simulink model "A1_finalized"  (R2024a)
settings: Solver=FixedStepAuto  StartTime=0.0  StopTime=10.0  FixedStep=1e-3  RelTol=1e-3  EnableMultiTasking=on
undefined symbols (not defined in the file): D0, D1, D10, D11, D12, D13, D2, D3, D4, D5, D6, D7, D8, D9, PTA0, PTA1, PTA2, PTB23, PTB9, PTC16, PTC17, PTC2, PTC3, PTC4, PTD0, PTD1, PTD2, PTD3
libraries: frdmk64flib x17
settings Model: ExtModeTrigDuration=5  Creator=haani  LastModifiedBy=hmz04
settings OptimizationCC: EnhancedBackFolding=on  PassReuseOutputArgsAs=Individual arguments  ZeroExternalMemoryAtStartup=off  ZeroInternalMemoryAtStartup=off  MaxStackSize=64  OptimizeBlockOrder=speed  DifferentSizesBufferReuse=on  OptimizationCustomize=off  EfficientTunableParamExpr=on
settings DebuggingCC: ParameterTunabilityLossMsg=error
settings HardwareCC: ProdBitPerPointer=32  ProdBitPerSizeT=32  ProdBitPerPtrDiffT=32  ProdLargestAtomicInteger=Long  ProdLargestAtomicFloat=Double  ProdWordSize=32  ProdHWDeviceType=ARM Compatible->ARM Cortex
settings SFSimCC: MATLABDynamicMemAlloc=off
settings RTWCC: Description=Embedded Coder  SystemTargetFile=ert.tlc  HardwareBoard=NXP FRDM-K64F  TLCOptions="-aInlineSetEventsForThisBaseRateFcn=TLC_FALSE -aSuppressMultiTaskScheduler=TLC_FALSE  -aRateBasedStepFcn=0"  TemplateMakefile=ert_default_tmf  Toolchain=GNU Tools for ARM Embedded Processors
settings CodeAppCC: ForceParamTrailComments=on  IgnoreCustomStorageClasses=off  OperatorAnnotations=on  SimulinkDataObjDesc=on  SFDataObjDesc=on  InsertBlockDesc=on
settings ERTTargetCC: ExtModeTransport=4  ExtModeMexFile=sendToCommService

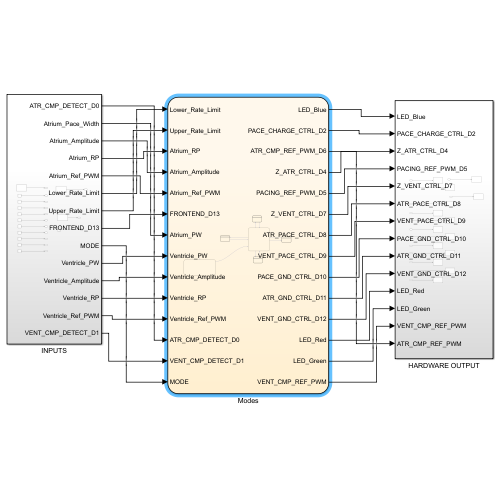
[thumbnail: Simulink's stored preview of the top-level diagram]
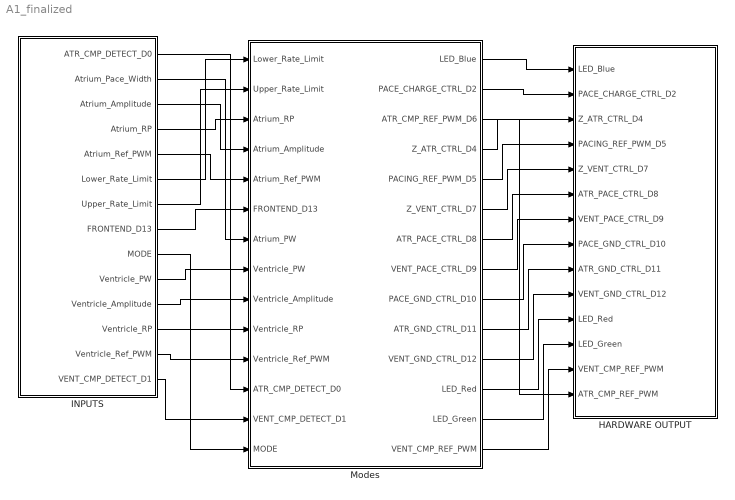
== system A1_finalized ==
  HARDWARE OUTPUT : Subsystem
  INPUTS : Subsystem
  Modes : Stateflow chart  TreatAsAtomicUnit=on
  wires:
  Modes/1(LED_Blue) -> HARDWARE OUTPUT/1(LED_Blue)
  Modes/2(PACE_CHARGE_CTRL_D2) -> HARDWARE OUTPUT/2(PACE_CHARGE_CTRL_D2)
  Modes/4(Z_ATR_CTRL_D4) -> HARDWARE OUTPUT/3(Z_ATR_CTRL_D4)
  Modes/5(PACING_REF_PWM_D5) -> HARDWARE OUTPUT/4(PACING_REF_PWM_D5)
  Modes/6(Z_VENT_CTRL_D7) -> HARDWARE OUTPUT/5(Z_VENT_CTRL_D7)
  Modes/7(ATR_PACE_CTRL_D8) -> HARDWARE OUTPUT/6(ATR_PACE_CTRL_D8)
  Modes/8(VENT_PACE_CTRL_D9) -> HARDWARE OUTPUT/7(VENT_PACE_CTRL_D9)
  Modes/9(PACE_GND_CTRL_D10) -> HARDWARE OUTPUT/8(PACE_GND_CTRL_D10)
  Modes/10(ATR_GND_CTRL_D11) -> HARDWARE OUTPUT/9(ATR_GND_CTRL_D11)
  Modes/11(VENT_GND_CTRL_D12) -> HARDWARE OUTPUT/10(VENT_GND_CTRL_D12)
  INPUTS/1(ATR_CMP_DETECT_D0) -> Modes/12(ATR_CMP_DETECT_D0)
  INPUTS/6(Lower_Rate_Limit) -> Modes/1(Lower_Rate_Limit)
  INPUTS/7(Upper_Rate_Limit) -> Modes/2(Upper_Rate_Limit)
  INPUTS/2(Atrium_Pace_Width) -> Modes/7(Atrium_PW)
  INPUTS/3(Atrium_Amplitude) -> Modes/4(Atrium_Amplitude)
  INPUTS/4(Atrium_RP) -> Modes/3(Atrium_RP)
  INPUTS/5(Atrium_Ref_PWM) -> Modes/5(Atrium_Ref_PWM)
  Modes/12(LED_Red) -> HARDWARE OUTPUT/11(LED_Red)
  Modes/13(LED_Green) -> HARDWARE OUTPUT/12(LED_Green)
  INPUTS/8(FRONTEND_D13) -> Modes/6(FRONTEND_D13)
  Modes/3(ATR_CMP_REF_PWM_D6) -> HARDWARE OUTPUT/14(ATR_CMP_REF_PWM)
  INPUTS/10(Ventricle_PW) -> Modes/8(Ventricle_PW)
  INPUTS/9(" MODE") -> Modes/14(MODE)
  INPUTS/11(Ventricle_Amplitude) -> Modes/9(Ventricle_Amplitude)
  INPUTS/12(Ventricle_RP) -> Modes/10(Ventricle_RP)
  INPUTS/13(Ventricle_Ref_PWM) -> Modes/11(Ventricle_Ref_PWM)
  INPUTS/14(VENT_CMP_DETECT_D1) -> Modes/13(VENT_CMP_DETECT_D1)
  Modes/14(VENT_CMP_REF_PWM) -> HARDWARE OUTPUT/13(VENT_CMP_REF_PWM)

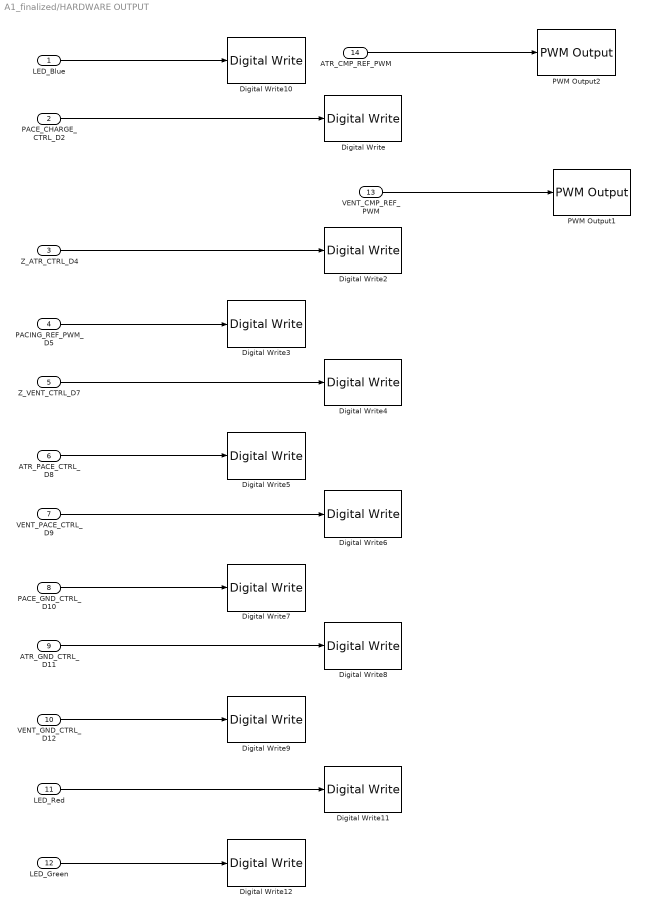
== system A1_finalized/HARDWARE OUTPUT ==
  LED_Blue : Inport
  PACE_CHARGE_CTRL_D2 : Inport  Port=2
  Z_ATR_CTRL_D4 : Inport  Port=3
  PACING_REF_PWM_D5 : Inport  Port=4
  Z_VENT_CTRL_D7 : Inport  Port=5
  ATR_PACE_CTRL_D8 : Inport  Port=6
  VENT_PACE_CTRL_D9 : Inport  Port=7
  PACE_GND_CTRL_D10 : Inport  Port=8
  ATR_GND_CTRL_D11 : Inport  Port=9
  VENT_GND_CTRL_D12 : Inport  Port=10
  LED_Red : Inport  Port=11
  LED_Green : Inport  Port=12
  VENT_CMP_REF_PWM : Inport  Port=13
  ATR_CMP_REF_PWM : Inport  Port=14
  Digital Write : frdmk64flib/Digital Write  Whichpin=PTB9 (D2)
  Digital Write10 : frdmk64flib/Digital Write  Whichpin=BLUE_LED
  Digital Write11 : frdmk64flib/Digital Write  Whichpin=RED_LED
  Digital Write12 : frdmk64flib/Digital Write  Whichpin=GREEN_LED
  Digital Write2 : frdmk64flib/Digital Write  Whichpin=PTB23 (D4)
  Digital Write3 : frdmk64flib/Digital Write  Whichpin=PTA2 (D5)
  Digital Write4 : frdmk64flib/Digital Write  Whichpin=PTC3 (D7)
  Digital Write5 : frdmk64flib/Digital Write  Whichpin=PTA0 (D8)
  Digital Write6 : frdmk64flib/Digital Write  Whichpin=PTC4 (D9)
  Digital Write7 : frdmk64flib/Digital Write  Whichpin=PTD0 (D10)
  Digital Write8 : frdmk64flib/Digital Write  Whichpin=PTD2 (D11)
  Digital Write9 : frdmk64flib/Digital Write  Whichpin=PTD3 (D12)
  PWM Output1 : frdmk64flib/PWM Output  Whichpin=PTA1 (D3)  InitialFrequency=2000  InitialDutyCycle=0
  PWM Output2 : frdmk64flib/PWM Output  Whichpin=PTC2 (D6)  InitialFrequency=2000  InitialDutyCycle=0
  wires:
  LED_Blue/1 -> Digital Write10/1
  PACE_CHARGE_CTRL_D2/1 -> Digital Write/1
  Z_ATR_CTRL_D4/1 -> Digital Write2/1
  PACING_REF_PWM_D5/1 -> Digital Write3/1
  Z_VENT_CTRL_D7/1 -> Digital Write4/1
  ATR_GND_CTRL_D11/1 -> Digital Write8/1
  PACE_GND_CTRL_D10/1 -> Digital Write7/1
  ATR_PACE_CTRL_D8/1 -> Digital Write5/1
  VENT_PACE_CTRL_D9/1 -> Digital Write6/1
  VENT_GND_CTRL_D12/1 -> Digital Write9/1
  LED_Green/1 -> Digital Write12/1
  LED_Red/1 -> Digital Write11/1
  VENT_CMP_REF_PWM/1 -> PWM Output1/1
  ATR_CMP_REF_PWM/1 -> PWM Output2/1

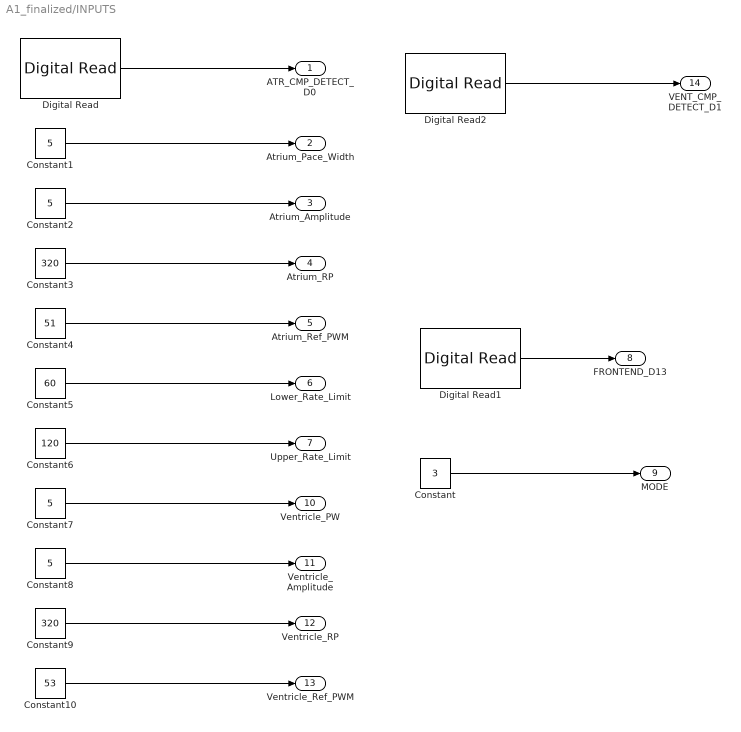
== system A1_finalized/INPUTS ==
  Constant : Constant  Value=3
  Constant{1..2,7..8} (4 alike) : Constant  Value=5  OutDataTypeStr=int16
  Constant10 : Constant  Value=53  OutDataTypeStr=int16
  Constant3 : Constant  Value=320  OutDataTypeStr=int16
  Constant4 : Constant  Value=51  OutDataTypeStr=int16
  Constant5 : Constant  Value=60  OutDataTypeStr=int16
  Constant6 : Constant  Value=120  OutDataTypeStr=int16
  Constant9 : Constant  Value=320  OutDataTypeStr=int16
  Digital Read : frdmk64flib/Digital Read  Whichpin=PTC16 (D0)  SampleTime=-1
  Digital Read1 : frdmk64flib/Digital Read  Whichpin=PTD1 (D13)  SampleTime=-1
  Digital Read2 : frdmk64flib/Digital Read  Whichpin=PTC17 (D1)  SampleTime=-1
  ATR_CMP_DETECT_D0 : Outport
  Atrium_Pace_Width : Outport  Port=2  OutDataTypeStr=int16
  Atrium_Amplitude : Outport  Port=3  OutDataTypeStr=int16
  Atrium_RP : Outport  Port=4  OutDataTypeStr=int16
  Atrium_Ref_PWM : Outport  Port=5  OutDataTypeStr=int16
  Lower_Rate_Limit : Outport  Port=6  OutDataTypeStr=int16
  Upper_Rate_Limit : Outport  Port=7  OutDataTypeStr=int16
  FRONTEND_D13 : Outport  Port=8
  " MODE" : Outport  Port=9
  Ventricle_PW : Outport  Port=10  OutDataTypeStr=int16
  Ventricle_Amplitude : Outport  Port=11  OutDataTypeStr=int16
  Ventricle_RP : Outport  Port=12  OutDataTypeStr=int16
  Ventricle_Ref_PWM : Outport  Port=13  OutDataTypeStr=int16
  VENT_CMP_DETECT_D1 : Outport  Port=14
  wires:
  Digital Read/1 -> ATR_CMP_DETECT_D0/1
  Constant1/1 -> Atrium_Pace_Width/1
  Constant2/1 -> Atrium_Amplitude/1
  Constant3/1 -> Atrium_RP/1
  Constant4/1 -> Atrium_Ref_PWM/1
  Constant5/1 -> Lower_Rate_Limit/1
  Constant6/1 -> Upper_Rate_Limit/1
  Digital Read1/1 -> FRONTEND_D13/1
  Constant/1 -> " MODE"/1
  Constant8/1 -> Ventricle_Amplitude/1
  Constant10/1 -> Ventricle_Ref_PWM/1
  Constant9/1 -> Ventricle_RP/1
  Constant7/1 -> Ventricle_PW/1
  Digital Read2/1 -> VENT_CMP_DETECT_D1/1

== stateflow chart A1_finalized/Modes ==
  state VVI
    state Refractory
      entry:
      PACING_REF_PWM_D5 = 100*(Ventricle_Amplitude/5)
      PACE_CHARGE_CTRL_D2=1;
      PACE_GND_CTRL_D10=1;
      VENT_PACE_CTRL_D9=0;
      Z_ATR_CTRL_D4=0;
      Z_VENT_CTRL_D7=0;
      ATR_PACE_CTRL_D8=0;
      ATR_GND_CTRL_D11=0;
      VENT_GND_CTRL_D12=1;
      VENT_CMP_REF_PWM= Ventricle_Ref_PWM;
      %Visual Signal
      LED_Blue=0;
      Period=60000/(Lower_Rate_Limit)
    state Pace
      entry:
      PACING_REF_PWM_D5=0
      PACE_CHARGE_CTRL_D2=0;
      PACE_GND_CTRL_D10=1;
      ATR_PACE_CTRL_D8=0;
      ATR_GND_CTRL_D11=0;
      Z_ATR_CTRL_D4=0;
      Z_VENT_CTRL_D7=0;
      VENT_GND_CTRL_D12=0;
      VENT_PACE_CTRL_D9=1;
      %Visual Signal
      LED_Blue=1;
      LED_Green=0;
    state Sense
      entry:
      LED_Green = 1;
    VVI.Pace -> VVI.Refractory : [after(Ventricle_PW,msec)]
    (default) -> VVI.Refractory
    VVI.Refractory -> VVI.Sense : [after(Ventricle_RP,msec)]
    VVI.Sense -> VVI.Pace [order 1] : [after(Period-Ventricle_RP-Ventricle_PW,msec)]
    VVI.Sense -> VVI.Refractory [order 2] : [VENT_CMP_DETECT_D1 == 1]
  state Mode
    %Reset everything
    entry:
    LED_Red  = 0;
    ATR_PACE_CTRL_D8 = 0;
    ATR_GND_CTRL_D11 = 0;
    VENT_GND_CTRL_D12 = 0;
    VENT_PACE_CTRL_D9 = 0;
    Z_ATR_CTRL_D4 = 0;
    Z_VENT_CTRL_D7 = 0;
    ATR_CMP_REF_PWM_D6 = 0;
    VENT_CMP_REF_PWM= 0;
    PACE_GND_CTRL_D10 = 0;
    PACE_CHARGE_CTRL_D2 = 0;
  state VOO
    state ChargeDischarge
      entry:
      %DISCHARGE C21 (resets everything)
      PACE_GND_CTRL_D10 = 1;
      ATR_GND_CTRL_D11 = 0;
      VENT_GND_CTRL_D12 = 1;
      VENT_PACE_CTRL_D9 = 0;
      ATR_PACE_CTRL_D8 = 0;
      Z_ATR_CTRL_D4 = 0;
      Z_VENT_CTRL_D7 = 0;
      %CHARGE C22 (prepare for next pulse)
      PACE_CHARGE_CTRL_D2=1;
      PACING_REF_PWM_D5 = Ventricle_Amplitude;
      %VISUAL SIGNAL
      LED_Blue = 0;
      %TIMING
      STANDBY_PERIOD = 30000/(Lower_Rate_Limit);
    state Pace1
      entry:
      %PROPER GND + TRIGGER PACE
      PACE_GND_CTRL_D10 = 1;
      ATR_GND_CTRL_D11 = 0;
      VENT_GND_CTRL_D12 = 0;
      VENT_PACE_CTRL_D9 = 1;
      ATR_PACE_CTRL_D8 = 0;
      Z_ATR_CTRL_D4 = 0;
      Z_VENT_CTRL_D7 = 0;
      PACE_CHARGE_CTRL_D2=0;
      PACING_REF_PWM_D5 = 0;
      %VISUAL SIGNAL
      LED_Blue = 1;
    (default) -> VOO.ChargeDischarge
    Pace1 -> VOO.ChargeDischarge : [after(Ventricle_PW,msec)]
    VOO.ChargeDischarge -> Pace1 : [after(STANDBY_PERIOD,msec)]
  state AAI
    state Pace
      entry:
      PACING_REF_PWM_D5=0
      PACE_CHARGE_CTRL_D2=0;
      PACE_GND_CTRL_D10=1;
      ATR_PACE_CTRL_D8=1;
      ATR_GND_CTRL_D11=0;
      Z_ATR_CTRL_D4=0;
      Z_VENT_CTRL_D7=0;
      VENT_GND_CTRL_D12=0;
      VENT_PACE_CTRL_D9=0;
      %Visual Signal
      LED_Blue=1;
      LED_Green = 0;
    state Refractory
      entry:
      PACING_REF_PWM_D5 = 100*(Atrium_Amplitude/5)
      PACE_CHARGE_CTRL_D2=1;
      PACE_GND_CTRL_D10=1;
      VENT_PACE_CTRL_D9=0;
      Z_ATR_CTRL_D4=0;
      Z_VENT_CTRL_D7=0;
      ATR_PACE_CTRL_D8=0;
      ATR_GND_CTRL_D11=1;
      VENT_GND_CTRL_D12=0;
      ATR_CMP_REF_PWM_D6= Atrium_Ref_PWM;
      %Visual Signal
      LED_Blue=0;
      Period=60000/(Lower_Rate_Limit)
    state Sense
      entry:
      LED_Green = 1;
    AAI.Pace -> AAI.Refractory : [after(Atrium_PW,msec)]
    (default) -> AAI.Refractory
    AAI.Refractory -> AAI.Sense : [after(Atrium_RP,msec)]
    AAI.Sense -> AAI.Pace [order 1] : [after(Period-Atrium_RP-Atrium_PW,msec)]
    AAI.Sense -> AAI.Refractory [order 2] : [ATR_CMP_DETECT_D0 == 1]
  state AOO
    state ChargeDischarge
      entry:
      %DISCHARGE C21 (resets everything)
      PACE_GND_CTRL_D10 = 1;
      ATR_GND_CTRL_D11 = 1;
      VENT_GND_CTRL_D12 = 0;
      VENT_PACE_CTRL_D9 = 0;
      ATR_PACE_CTRL_D8 = 0;
      Z_ATR_CTRL_D4 = 0;
      Z_VENT_CTRL_D7 = 0;
      %CHARGE C22 (prepare for next pulse)
      PACE_CHARGE_CTRL_D2=1;
      PACING_REF_PWM_D5 = Atrium_Amplitude;
      %VISUAL SIGNAL
      LED_Blue = 0;
      %TIMING
      STANDBY_PERIOD = 30000/(Lower_Rate_Limit);
    state Pace
      entry:
      %PROPER GND + TRIGGER PACE
      PACE_GND_CTRL_D10 = 1;
      ATR_GND_CTRL_D11 = 0;
      VENT_GND_CTRL_D12 = 0;
      VENT_PACE_CTRL_D9 = 0;
      ATR_PACE_CTRL_D8 = 1;
      Z_ATR_CTRL_D4 = 0;
      Z_VENT_CTRL_D7 = 0;
      PACE_CHARGE_CTRL_D2=0;
      PACING_REF_PWM_D5 = 0;
      %VISUAL SIGNAL
      LED_Blue = 1;
    (default) -> AOO.ChargeDischarge
    AOO.Pace -> AOO.ChargeDischarge : [after(Atrium_PW,msec)]
    AOO.ChargeDischarge -> AOO.Pace : [after(STANDBY_PERIOD,msec)]
  state Safety
    %LED turns red if any of the user input values are unsafe
    entry:
    LED_Red = 1;
  Mode -> VVI [order 4] : [MODE==3]
  VVI -> Mode : [MODE~=3]
  Mode -> VOO [order 2] : [MODE==2]
  AAI -> Mode : [MODE~=4]
  VOO -> Mode : [MODE~=2]
  Mode -> AAI [order 3] : [MODE==4]
  Safety -> Mode : [Lower_Rate_Limit < 175 && Atrium_Amplitude < 7 && Ventricle_Amplitude < 7  && Atrium_RP <= 500 && Ventricle_RP <= 500 && Atrium_RP >= 150 && Ventricle_RP >= 150]
  Mode -> AOO [order 1] : [MODE==1]
  AOO -> Mode : [MODE~=1]
  (default) -> Safety
  data: LED_Blue output double; PACE_CHARGE_CTRL_D2 output double; ATR_CMP_REF_PWM_D6 output int16; Z_ATR_CTRL_D4 output double; PACING_REF_PWM_D5 output int16; Z_VENT_CTRL_D7 output double; ATR_PACE_CTRL_D8 output double; VENT_PACE_CTRL_D9 output double; PACE_GND_CTRL_D10 output double; ATR_GND_CTRL_D11 output double; VENT_GND_CTRL_D12 output double; Lower_Rate_Limit input int16; Upper_Rate_Limit input int16; Atrium_RP input int16; Atrium_Amplitude input int16; Atrium_Ref_PWM input; FRONTEND_D13 input; Atrium_PW input int16; Ventricle_PW input; Ventricle_Amplitude input; Ventricle_RP input; Ventricle_Ref_PWM input; ATR_CMP_DETECT_D0 input; VENT_CMP_DETECT_D1 input; LED_Red output double; LED_Green output double; Standby_Period local; MODE input; Period local; STANDBY_PERIOD local; VENT_CMP_REF_PWM output
